simulink model "Subsystem"  (R2020b)
settings: Solver=FixedStepAuto  StartTime=0.0  StopTime=50  FixedStep=1  RelTol=1e-3
settings Model: Creator=baner  LastModifiedBy=baner
settings DataIOCC: SaveOutput=off  SaveTime=off

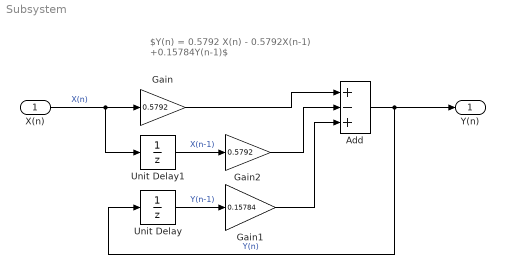
== system Subsystem ==
  note: $Y(n) = 0.5792 X(n) - 0.5792X(n-1) +0.15784Y(n-1)$
  X(n) : Inport  OutDataTypeStr=double  PortDimensions=1  SampleTime=[1,0]
  Add : Sum  Inputs=+-+
  Gain : Gain  Gain=0.5792
  Gain1 : Gain  Gain=0.15784
  Gain2 : Gain  Gain=0.5792
  Unit Delay : UnitDelay  SampleTime=-1  HasFrameUpgradeWarning=on
  Unit Delay1 : UnitDelay  SampleTime=-1  HasFrameUpgradeWarning=on
  Y(n) : Outport  OutDataTypeStr=double  PortDimensions=1  SampleTime=[1,0]
  wires:
  Unit Delay/1 -> Gain1/1  "Y(n-1)"
  Gain/1 -> Add/1
  Gain1/1 -> Add/3
  X(n)/1 -> Gain/1, Unit Delay1/1  "X(n)"
  Unit Delay1/1 -> Gain2/1  "X(n-1)"
  Gain2/1 -> Add/2
  Add/1 -> Unit Delay/1, Y(n)/1  "Y(n)"
